simulink model "Active_suspension_model_simulation"  (R2017b)
settings: Solver=ode4  StartTime=0.0  StopTime=10.00  FixedStep=0.001  RelTol=1e-3  EnableMultiTasking=on
libraries: simulink x1
settings Model: Creator=Shrey Jain  LastModifiedBy=Shrey Jain
settings DataIOCC: LimitDataPoints=on  SaveFormat=Array
settings OptimizationCC: LifeSpan=inf
settings DebuggingCC: SFUnexpectedBacktrackingDiag=warning  SFNoUnconditionalDefaultTransitionDiag=warning  SFExecutionAtInitializationDiag=none
settings HardwareCC: ProdBitPerPointer=32  ProdBitPerSizeT=32  ProdBitPerPtrDiffT=32  ProdLargestAtomicFloat=None  ProdIntDivRoundTo=Undefined  ProdEndianess=Unspecified  ProdWordSize=32  ProdHWDeviceType=32-bit Generic
settings ModelReferenceCC: PropagateSignalLabelsOutOfModel=off
settings CodeAppCC: StateflowObjectComments=on
settings GRTTargetCC: TargetLangStandard=C89/C90 (ANSI)  GeneratePreprocessorConditionals=Disable all
settings ConfigComp: CovMetricSettings=dw  CovHtmlReporting=on  CovSaveCumulativeToWorkspaceVar=on  CovSaveSingleToWorkspaceVar=on  CovExternalEMLEnable=off

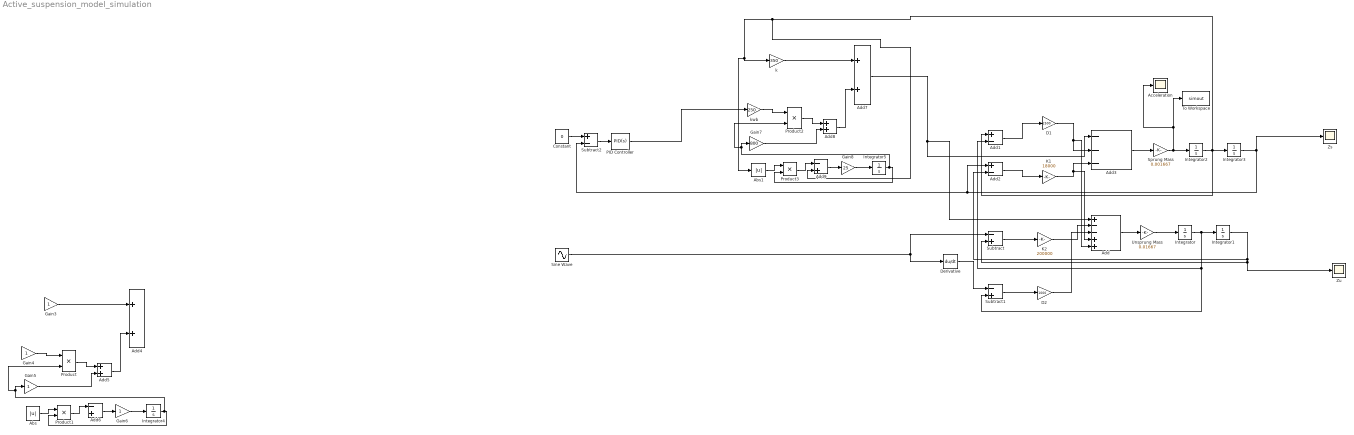
== system Active_suspension_model_simulation ==
  Abs : Abs
  Abs1 : Abs
  Acceleration : Scope
  Add : Sum  Inputs=+--++
  Add1 : Sum  Inputs=+-
  Add2 : Sum  Inputs=+-
  Add3 : Sum  Inputs=---
  Add{4..5,7..8} (4 alike) : Sum
  Add6 : Sum  Inputs=-+
  Add9 : Sum  Inputs=-+
  Constant : Constant  Value=0
  D1 : Gain  Gain=2500
  D2 : Gain  Gain=1000
  Derivative : Derivative
  Gain{3..6} (4 alike) : Gain
  Gain7 : Gain  Gain=800
  Gain8 : Gain  Gain=25
  Integrator{,1..5} (6 alike) : Integrator
  K1 : Gain  Gain=18000
  K2 : Gain  Gain=200000
  PID Controller : simulink/Continuous/PID Controller  Controller=PID  TimeDomain=Continuous-time  SampleTime=-1  IntegratorMethod=Forward Euler  FilterMethod=Forward Euler  Form=Parallel  UseFilter=on  ControllerParametersSource=internal  P=10  I=5  D=15  N=100  InitialConditionSource=internal  InitialConditionForIntegrator=0  InitialConditionForFilter=0  ExternalReset=none  LimitOutput=off  UpperSaturationLimit=inf  LowerSaturationLimit=-inf  LinearizeAsGain=on  AntiWindupMode=none  Kb=1  TrackingMode=off  Kt=1  PParamMin=[]  PParamMax=[]  IParamMin=[]  IParamMax=[]  DParamMin=[]  DParamMax=[]  NParamMin=[]  NParamMax=[]  KbParamMin=[]  KbParamMax=[]  KtParamMin=[]  KtParamMax=[]  POutMin=[]  POutMax=[]  IOutMin=[]  IOutMax=[]  DOutMin=[]  DOutMax=[]  NOutMin=[]  NOutMax=[]  KbOutMin=[]  KbOutMax=[]  KtOutMin=[]  KtOutMax=[]  IntegratorOutMin=[]  IntegratorOutMax=[]  FilterOutMin=[]  FilterOutMax=[]  SumOutMin=[]  SumOutMax=[]  SumI1OutMin=[]  SumI1OutMax=[]  SumI2OutMin=[]  SumI2OutMax=[]  SumI3OutMin=[]  SumI3OutMax=[]  SumDOutMin=[]  SumDOutMax=[]  SaturationOutMin=[]  SaturationOutMax=[]  IntegratorContinuousStateAttributes=''  IntegratorStateMustResolveToSignalObject=off  IntegratorRTWStateStorageClass=Auto  FilterContinuousStateAttributes=''  FilterStateMustResolveToSignalObject=off  FilterRTWStateStorageClass=Auto  DifferentiatorICPrevScaledInput=0  DifferentiatorOutMin=[]  DifferentiatorOutMax=[]  InitialConditionSetting=State (most efficient)  FilterDiffOutCoefMin=[]  FilterDiffOutCoefMax=[]  SumDenOutMin=[]  SumDenOutMax=[]  SumNumOutMin=[]  SumNumOutMax=[]  ReciprocalOutMin=[]  ReciprocalOutMax=[]  DivideOutMin=[]  DivideOutMax=[]  TunerSelectOption=Transfer Function Based (PID Tuner App)
  Product{,1..3} (4 alike) : Product
  Sine Wave : Sin  Frequency=2*pi  SampleTime=0
  Sprung Mass : Gain  Gain=0.001667
  Subtract : Sum  Inputs=-+
  Subtract1 : Sum  Inputs=-+
  Subtract2 : Sum  Inputs=+-
  To Workspace : ToWorkspace  VariableName=simout  SampleTime=-1
      settings: Save2DSignal=2-D array (concatenate along first dimension)
  Unsprung Mass : Gain  Gain=0.01667
  Zs : Scope
  Zu : Scope
  k : Gain  Gain=350
  kwb : Gain  Gain=250
  wires:
  Sprung Mass/1 -> Acceleration/1, To Workspace/1, Integrator2/1
  Integrator3/1 -> Zs/1, Subtract2/2, Add2/1
  Integrator1/1 -> Zu/1, Subtract/2, Add2/2
  Derivative/1 -> Subtract1/1
  Add/1 -> Unsprung Mass/1
  D2/1 -> Add/3
  D1/1 -> Add/5, Add3/2
  K2/1 -> Add/2
  Add3/1 -> Sprung Mass/1
  Add7/1 -> Add3/1, Add/1
  Subtract/1 -> K2/1
  Unsprung Mass/1 -> Integrator/1
  Sine Wave/1 -> Derivative/1, Subtract/1
  K1/1 -> Add/4, Add3/3
  Constant/1 -> Subtract2/1
  Add1/1 -> D1/1
  Subtract1/1 -> D2/1
  Add2/1 -> K1/1
  Integrator/1 -> Add1/2, Subtract1/2, Integrator1/1
  Gain4/1 -> Product/1
  Gain5/1 -> Add5/2
  Product/1 -> Add5/1
  Gain3/1 -> Add4/1
  Add5/1 -> Add4/2
  Add6/1 -> Gain6/1
  Abs/1 -> Product1/1
  Integrator4/1 -> Product/2, Gain5/1, Product1/2
  Product1/1 -> Add6/1
  Gain6/1 -> Integrator4/1
  Subtract2/1 -> PID Controller/1
  Product3/1 -> Add9/1
  Add9/1 -> Gain8/1
  Gain7/1 -> Add8/2
  Gain8/1 -> Integrator5/1
  Abs1/1 -> Product3/1
  k/1 -> Add7/1
  Integrator5/1 -> Product2/2, Gain7/1, Product3/2
  Product2/1 -> Add8/1
  kwb/1 -> Product2/1
  Add8/1 -> Add7/2
  Integrator2/1 -> Add9/2, Abs1/1, k/1, Add1/1, Integrator3/1
  PID Controller/1 -> kwb/1
